simulink library "sensor_conversion_blocks"  (R2025b)
settings: Solver=VariableStepAuto  StartTime=0.0  StopTime=10.0  RelTol=1e-3
undefined symbols (not defined in the file): D
libraries: slrealtimeloglib x7, dspsigattribs x6, dspstat3 x5, dspfdesign x4, dspswit3 x2, eeGeneralControl x1
settings Model: Creator=cmmcguir  LastModifiedBy=cmmcguir

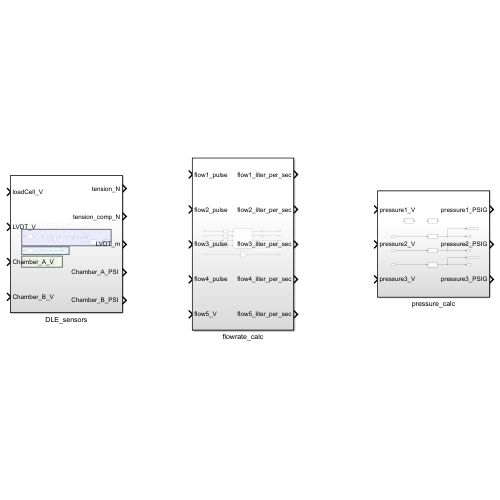
[thumbnail: Simulink's stored preview of the top-level diagram]
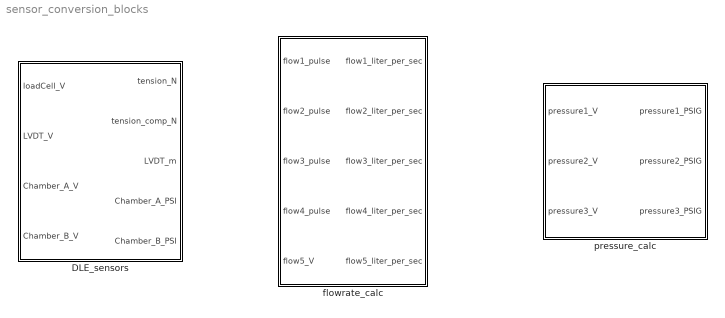
== system sensor_conversion_blocks ==
  DLE_sensors : Subsystem
  flowrate_calc : Subsystem
  pressure_calc : Subsystem

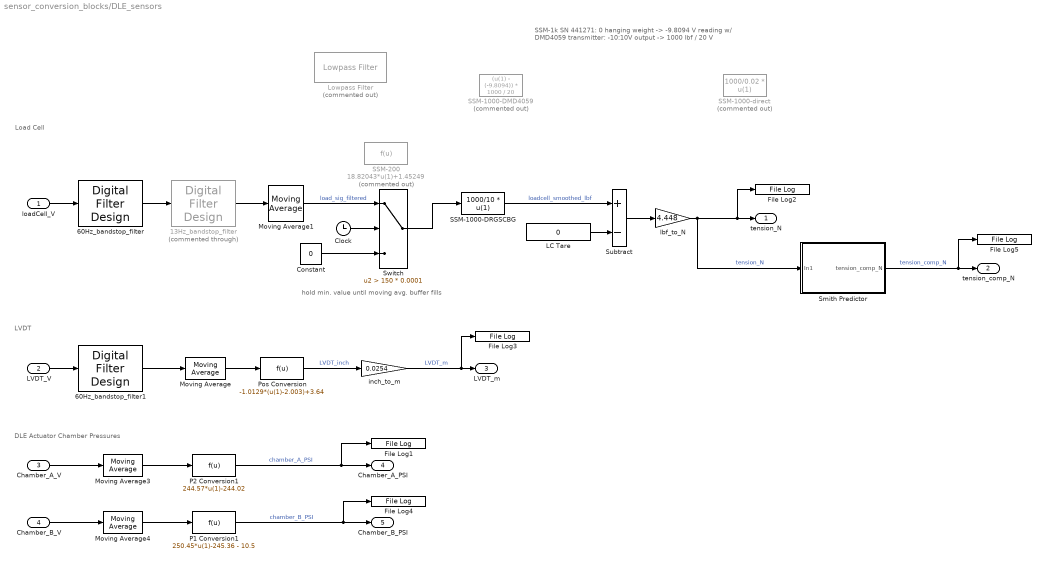
== system sensor_conversion_blocks/DLE_sensors ==
  note: hold min. value until moving avg. buffer fills
  note: SSM-1k SN 441271: 0 hanging weight -> -9.8094 V reading
      | w/ DMD4059 transmitter: -10:10V output -> 1000 lbf  / 20 V
  note: DLE Actuator Chamber Pressures
  note: LVDT
  note: Load Cell
  loadCell_V : Inport
  LVDT_V : Inport  Port=2
  Chamber_A_V : Inport  Port=3
  Chamber_B_V : Inport  Port=4
  13Hz_bandstop_filter : dspfdesign/Digital Filter Design  Commented=through  mwdsp_browser_bugfix_var=off
  60Hz_bandstop_filter : dspfdesign/Digital Filter Design  mwdsp_browser_bugfix_var=off
  60Hz_bandstop_filter1 : dspfdesign/Digital Filter Design  mwdsp_browser_bugfix_var=off
  Clock : Clock
  Constant : Constant  Value=0
  File Log{1..5} (5 alike) : slrealtimeloglib/File Log  decimation=1  inputProcessing=Elements as channels (sample based)
  LC Tare : Constant  Value=0
  Lowpass Filter : dspfdesign/Lowpass Filter  Commented=on  FilterType=FIR  DesignForMinimumOrder=on  FilterOrder=50  PassbandFrequency=10  StopbandFrequency=250  PassbandRipple=0.1  StopbandAttenuation=80  SampleRateMode=Specify on dialog  SampleRate=10000  SimulateUsing=Interpreted execution  roundingMode=Floor  coeffsDataTypeStr=fixdt(1,16)
  Moving Average : dspstat3/Moving Average  Method=Sliding window  ForgettingFactorPort=off  SpecifyWindowLength=on  WindowLength=150  OverlapLength=149  AllowArbitraryInputLength=off  ForgettingFactor=0.1  SimulateUsing=Code generation
  Moving Average1 : dspstat3/Moving Average  Method=Sliding window  ForgettingFactorPort=off  SpecifyWindowLength=on  WindowLength=150  OverlapLength=149  AllowArbitraryInputLength=off  ForgettingFactor=0.9  SimulateUsing=Interpreted execution
  Moving Average3 : dspstat3/Moving Average  Method=Sliding window  ForgettingFactorPort=off  SpecifyWindowLength=on  WindowLength=100  OverlapLength=99  AllowArbitraryInputLength=off  ForgettingFactor=0.1  SimulateUsing=Code generation
  Moving Average4 : dspstat3/Moving Average  Method=Sliding window  ForgettingFactorPort=off  SpecifyWindowLength=on  WindowLength=100  OverlapLength=99  AllowArbitraryInputLength=off  ForgettingFactor=0.1  SimulateUsing=Code generation
  P1 Conversion1 : Fcn  Expr=250.45*u(1)-245.36 - 10.5
  P2 Conversion1 : Fcn  Expr=244.57*u(1)-244.02
  Pos Conversion : Fcn  Expr=-1.0129*(u(1)-2.003)+3.64
  SSM-1000-DMD4059 : Fcn  Commented=on  Expr=(u(1) - (-9.8094)) * 1000 / 20
  SSM-1000-DRGSCBG : Fcn  Expr=1000/10 * u(1)
  SSM-1000-direct : Fcn  Commented=on  Expr=1000/0.02 * u(1)
  SSM-200 : Fcn  Commented=on  Expr=18.82043*u(1)+1.45249
  Smith Predictor : Subsystem
  Subtract : Sum  Inputs=+-
  Switch : Switch  Criteria=u2 > Threshold  Threshold=150 * 0.0001  SaturateOnIntegerOverflow=off  InputSameDT=off
  inch_to_m : Gain  Gain=0.0254
  lbf_to_N : Gain  Gain=4.448
  tension_N : Outport
  tension_comp_N : Outport  Port=2
  LVDT_m : Outport  Port=3
  "Chamber_A_PSI " : Outport  Port=4  VectorParamsAs1DForOutWhenUnconnected=off
  "Chamber_B_PSI " : Outport  Port=5  VectorParamsAs1DForOutWhenUnconnected=off
  wires:
  SSM-1000-DRGSCBG/1 -> Subtract/1  "loadcell_smoothed_lbf"
  LC Tare/1 -> Subtract/2
  Subtract/1 -> lbf_to_N/1
  lbf_to_N/1 -> Smith Predictor/1(In1), File Log2/1, tension_N/1  "tension_N"
  Pos Conversion/1 -> inch_to_m/1  "LVDT_inch"
  inch_to_m/1 -> File Log3/1, LVDT_m/1  "LVDT_m"
  60Hz_bandstop_filter/1 -> 13Hz_bandstop_filter/1
  13Hz_bandstop_filter/1 -> Moving Average1/1
  LVDT_V/1 -> 60Hz_bandstop_filter1/1
  60Hz_bandstop_filter1/1 -> Moving Average/1
  Moving Average/1 -> Pos Conversion/1
  P2 Conversion1/1 -> File Log1/1, "Chamber_A_PSI "/1  "chamber_A_PSI"
  P1 Conversion1/1 -> File Log4/1, "Chamber_B_PSI "/1  "chamber_B_PSI"
  Chamber_B_V/1 -> Moving Average4/1
  Chamber_A_V/1 -> Moving Average3/1
  Moving Average3/1 -> P2 Conversion1/1
  Moving Average4/1 -> P1 Conversion1/1
  Smith Predictor/1(tension_comp_N) -> File Log5/1, tension_comp_N/1  "tension_comp_N"
  Switch/1 -> SSM-1000-DRGSCBG/1
  Clock/1 -> Switch/2
  Constant/1 -> Switch/3
  loadCell_V/1 -> 60Hz_bandstop_filter/1
  Moving Average1/1 -> Switch/1  "load_sig_filtered"

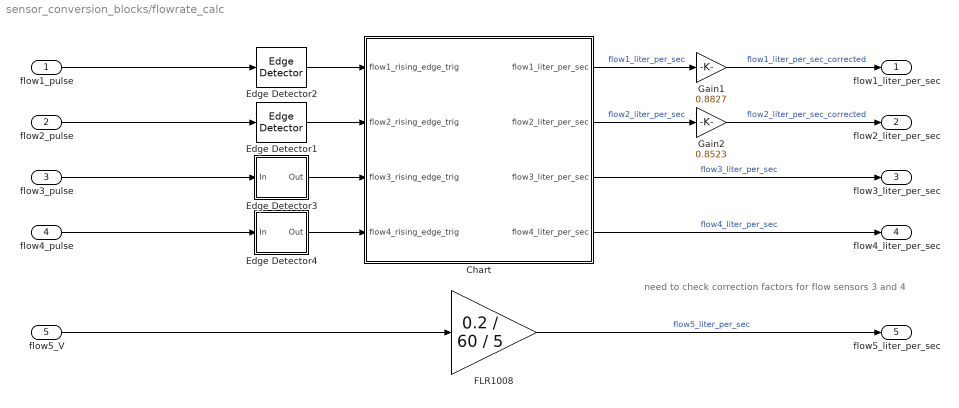
== system sensor_conversion_blocks/flowrate_calc ==
  note: need to check correction factors for flow sensors 3 and 4
  flow1_pulse : Inport
  flow2_pulse : Inport  Port=2
  flow3_pulse : Inport  Port=3
  flow4_pulse : Inport  Port=4
  flow5_V : Inport  Port=5
  Chart : Stateflow chart  TreatAsAtomicUnit=on
  Edge Detector1 : dspswit3/Edge Detector  InputProcessing=Columns as channels (frame based)
  Edge Detector2 : dspswit3/Edge Detector  InputProcessing=Columns as channels (frame based)
  Edge Detector3 : Subsystem  mask(Edge Detector){InputProcessing=Columns as channels (frame based)}
      mask prompts: InputProcessing "dsp:FIRMultirateBlockDialog:InputProc_MP"
      mask help: dsp:DSPSwitchesBlockDialog:EdgeDetector_MaskDesc
      mask init:
      | inputProc = get_param(gcbh, 'InputProcessing');
      | set_param([gcb '/Delay'], 'InputProcessing', inputProc);
      mask Help: eval('blocksethelp');
      mask TypeOptions InputProcessing: dsp:dialog:InProcessingFrameBased_CB | dsp:dialog:InProcessingSampleBased_CB
      mask DialogControl InputProcessing Prompt: Input processing:
      mask Display:
      | x = [.1 .2 .2 .5 .5 .7 .7 .8 .8 .9 NaN .1 .9 NaN .2 .2 NaN .7 .7];
      | y = [.6 .6 .9 .9 .6 .6 .9 .9 .6 .6 NaN .1 .1 NaN .1 .5 NaN .1 .5];
      | plot(x,y)
  Edge Detector4 : Subsystem  mask(Edge Detector){InputProcessing=Columns as channels (frame based)}
      mask prompts: InputProcessing "dsp:FIRMultirateBlockDialog:InputProc_MP"
      mask help: dsp:DSPSwitchesBlockDialog:EdgeDetector_MaskDesc
      mask init:
      | inputProc = get_param(gcbh, 'InputProcessing');
      | set_param([gcb '/Delay'], 'InputProcessing', inputProc);
      mask Help: eval('blocksethelp');
      mask TypeOptions InputProcessing: dsp:dialog:InProcessingFrameBased_CB | dsp:dialog:InProcessingSampleBased_CB
      mask DialogControl InputProcessing Prompt: Input processing:
      mask Display:
      | x = [.1 .2 .2 .5 .5 .7 .7 .8 .8 .9 NaN .1 .9 NaN .2 .2 NaN .7 .7];
      | y = [.6 .6 .9 .9 .6 .6 .9 .9 .6 .6 NaN .1 .1 NaN .1 .5 NaN .1 .5];
      | plot(x,y)
  FLR1008 : Gain  Gain=0.2 / 60 / 5
  Gain1 : Gain  Gain=0.8827
  Gain2 : Gain  Gain=0.8523
  flow1_liter_per_sec : Outport
  flow2_liter_per_sec : Outport  Port=2
  flow3_liter_per_sec : Outport  Port=3
  flow4_liter_per_sec : Outport  Port=4
  flow5_liter_per_sec : Outport  Port=5
  wires:
  flow2_pulse/1 -> Edge Detector1/1
  Edge Detector1/1 -> Chart/2(flow2_rising_edge_trig)
  Chart/1(flow1_liter_per_sec) -> Gain1/1  "flow1_liter_per_sec"
  Chart/2(flow2_liter_per_sec) -> Gain2/1  "flow2_liter_per_sec"
  flow1_pulse/1 -> Edge Detector2/1
  Edge Detector2/1 -> Chart/1(flow1_rising_edge_trig)
  Gain1/1 -> flow1_liter_per_sec/1  "flow1_liter_per_sec_corrected"
  Gain2/1 -> flow2_liter_per_sec/1  "flow2_liter_per_sec_corrected"
  flow3_pulse/1 -> Edge Detector3/1(In)
  flow4_pulse/1 -> Edge Detector4/1(In)
  Edge Detector3/1(Out) -> Chart/3(flow3_rising_edge_trig)
  Edge Detector4/1(Out) -> Chart/4(flow4_rising_edge_trig)
  Chart/3(flow3_liter_per_sec) -> flow3_liter_per_sec/1  "flow3_liter_per_sec"
  Chart/4(flow4_liter_per_sec) -> flow4_liter_per_sec/1  "flow4_liter_per_sec"
  flow5_V/1 -> FLR1008/1
  FLR1008/1 -> flow5_liter_per_sec/1  "flow5_liter_per_sec"

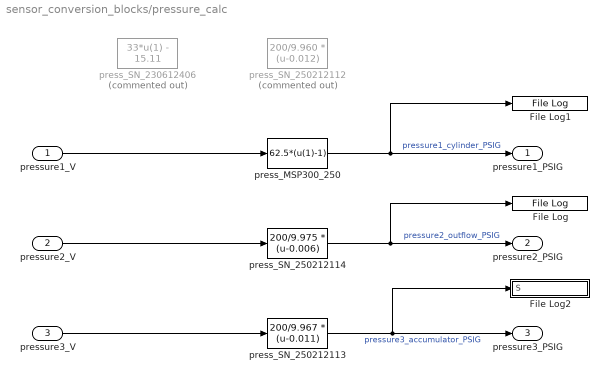
== system sensor_conversion_blocks/pressure_calc ==
  pressure1_V : Inport
  pressure2_V : Inport  Port=2
  pressure3_V : Inport  Port=3
  File Log : slrealtimeloglib/File Log  decimation=1  inputProcessing=Elements as channels (sample based)
  File Log1 : slrealtimeloglib/File Log  decimation=1  inputProcessing=Elements as channels (sample based)
  File Log2 : Subsystem  mask(slrealtimeloggingblock){decimation=1, inputProcessing=Elements as channels (sample based)}
      mask prompts: decimation "slrealtime:maskStrings:Decimation"; inputProcessing "slrealtime:maskStrings:InputProcessing"
      mask help: slrealtime:maskStrings:FileLogDesc
      mask init:
      | slrealtime.internal.logging.mloggingblock(gcb, decimation, inputProcessing);
      mask Help: eval('slrealtimedoc(''File_Log'')');
      mask TypeOptions inputProcessing: slrealtime:maskStrings:FrameBased | slrealtime:maskStrings:SampleBased
      mask DialogControl DescGroupVar Prompt: File Log
      mask DialogControl decimation Prompt: Decimation
      mask DialogControl inputProcessing Prompt: Input Processing
      mask Display: fprintf(message('slrealtime:maskStrings:FileLogDisp').getString);
  press_MSP300_250 : Fcn  Expr=62.5*(u(1)-1)
  press_SN_230612406 : Fcn  Commented=on  Expr=33*u(1) - 15.11
  press_SN_250212112 : Fcn  Commented=on  Expr=200/9.960 * (u-0.012)
  press_SN_250212113 : Fcn  Expr=200/9.967 * (u-0.011)
  press_SN_250212114 : Fcn  Expr=200/9.975 * (u-0.006)
  pressure1_PSIG : Outport
  pressure2_PSIG : Outport  Port=2
  pressure3_PSIG : Outport  Port=3
  wires:
  pressure1_V/1 -> press_MSP300_250/1
  press_MSP300_250/1 -> pressure1_PSIG/1, File Log1/1  "pressure1_cylinder_PSIG"
  press_SN_250212114/1 -> pressure2_PSIG/1, File Log/1  "pressure2_outflow_PSIG"
  pressure2_V/1 -> press_SN_250212114/1
  pressure3_V/1 -> press_SN_250212113/1
  press_SN_250212113/1 -> File Log2/1(S), pressure3_PSIG/1  "pressure3_accumulator_PSIG"

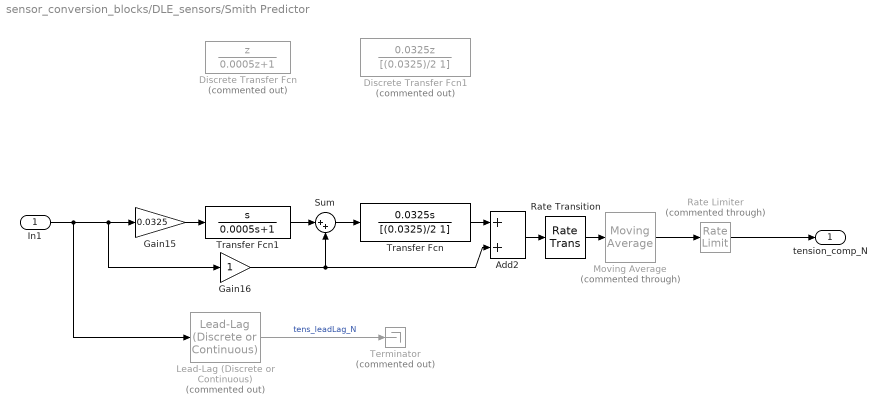
== system sensor_conversion_blocks/DLE_sensors/Smith Predictor ==
  In1 : Inport
  Add2 : Sum
  Discrete Transfer Fcn : DiscreteTransferFcn  Commented=on  Numerator=[1 0]  Denominator=[0.0005 1]
  Discrete Transfer Fcn1 : DiscreteTransferFcn  Commented=on  Numerator=[0.0325 0]  Denominator=[(0.0325)/2 1]
  Gain15 : Gain  Gain=0.0325
  Gain16 : Gain
  Lead-Lag (Discrete or Continuous) : eeGeneralControl/Lead-Lag (Discrete or Continuous)  Commented=on  T1=0.3  T2=0.1  B=inf  A=-inf  init_option=Inherited from block input  x0=0  Ts=-1
      settings: LibrarySourceBlock=|
      | ee_sl_lib/General Control/Lead-Lag
      | (Discrete or Continuous)
  Moving Average : dspstat3/Moving Average  Commented=through  Method=Sliding window  ForgettingFactorPort=off  SpecifyWindowLength=on  WindowLength=50  OverlapLength=49  AllowArbitraryInputLength=off  ForgettingFactor=0.9  SimulateUsing=Interpreted execution
  Rate Limiter : RateLimiter  Commented=through  RisingSlewLimit=4e3  FallingSlewLimit=-4e3  SampleTimeMode=inherited
  Rate Transition : RateTransition  OutPortSampleTime=0.0001
  Sum : Sum  Inputs=|++
  Terminator : Terminator  Commented=on
  Transfer Fcn : TransferFcn  Numerator=[0.0325 0]  Denominator=[(0.0325)/2 1]
  Transfer Fcn1 : TransferFcn  Numerator=[1 0]  Denominator=[0.0005 1]
  tension_comp_N : Outport
  wires:
  Gain16/1 -> Sum/2, Add2/2
  Transfer Fcn1/1 -> Sum/1
  In1/1 -> Lead-Lag (Discrete or Continuous)/1, Gain15/1, Gain16/1
  Gain15/1 -> Transfer Fcn1/1
  Add2/1 -> Rate Transition/1
  Sum/1 -> Transfer Fcn/1
  Transfer Fcn/1 -> Add2/1
  Moving Average/1 -> Rate Limiter/1
  Rate Transition/1 -> Moving Average/1
  Lead-Lag (Discrete or Continuous)/1 -> Terminator/1  "tens_leadLag_N"
  Rate Limiter/1 -> tension_comp_N/1

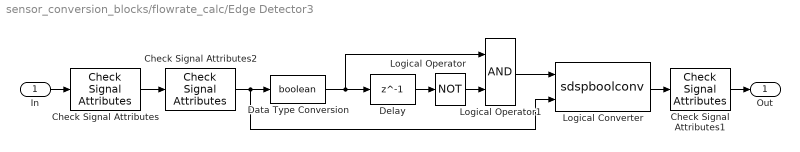
== system sensor_conversion_blocks/flowrate_calc/Edge Detector3 ==
  In : Inport
  Check Signal Attributes : dspsigattribs/Check Signal Attributes  SigAttribCheckMethod=Matches attributes exactly  Complexity=Ignore  Frame=Ignore  DimsCheckMethod=Ignore  Dimensions=1-D  DatatypeCheckMethod=Is...  DatatypeGeneral=Enumerated  DtypeFloatSpecific=Any floating-point  DtypeFixedSpecific=Any fixed-point  DtypeIntSpecific=Any integer  SampleMode=Ignore
  Check Signal Attributes1 : dspsigattribs/Check Signal Attributes  SigAttribCheckMethod=Matches attributes exactly  Complexity=Ignore  Frame=Ignore  DimsCheckMethod=Ignore  Dimensions=1-D  DatatypeCheckMethod=Is...  DatatypeGeneral=Enumerated  DtypeFloatSpecific=Any floating-point  DtypeFixedSpecific=Any fixed-point  DtypeIntSpecific=Any integer  SampleMode=Ignore
  Check Signal Attributes2 : dspsigattribs/Check Signal Attributes  SigAttribCheckMethod=Matches attributes exactly  Complexity=Ignore  Frame=Ignore  DimsCheckMethod=Ignore  Dimensions=1-D  DatatypeCheckMethod=Ignore  DatatypeGeneral=Enumerated  DtypeFloatSpecific=Any floating-point  DtypeFixedSpecific=Any fixed-point  DtypeIntSpecific=Any integer  SampleMode=Continuous
  Data Type Conversion : DataTypeConversion  OutDataTypeStr=boolean
  Delay : Delay  DelayLength=1  InitialCondition=1  InputProcessing=Columns as channels (frame based)
  Logical Operator : Logic  Operator=NOT  Inputs=1
  Logical Operator1 : Logic
  Logical Converter : S-Function  FunctionName=sdspboolconv  SFunctionDeploymentMode=off  EnableBusSupport=off
      mask Display:
      | disp('Logical\nConverter');
      | 
      | 
      | 
      | 
      | 
      | port_label('input',1, 'In');
      | 
      | 
      | 
      | 
      | 
      | port_label('input',2, 'Ref');
  Out : Outport  InitialOutput=0
  wires:
  Logical Operator1/1 -> Logical Converter/1
  Logical Operator/1 -> Logical Operator1/2
  Data Type Conversion/1 -> Logical Operator1/1, Delay/1
  Delay/1 -> Logical Operator/1
  In/1 -> Check Signal Attributes/1
  Logical Converter/1 -> Check Signal Attributes1/1
  Check Signal Attributes/1 -> Check Signal Attributes2/1
  Check Signal Attributes1/1 -> Out/1
  Check Signal Attributes2/1 -> Logical Converter/2, Data Type Conversion/1

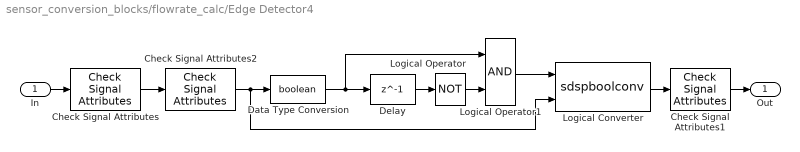
== system sensor_conversion_blocks/flowrate_calc/Edge Detector4 ==
  In : Inport
  Check Signal Attributes : dspsigattribs/Check Signal Attributes  SigAttribCheckMethod=Matches attributes exactly  Complexity=Ignore  Frame=Ignore  DimsCheckMethod=Ignore  Dimensions=1-D  DatatypeCheckMethod=Is...  DatatypeGeneral=Enumerated  DtypeFloatSpecific=Any floating-point  DtypeFixedSpecific=Any fixed-point  DtypeIntSpecific=Any integer  SampleMode=Ignore
  Check Signal Attributes1 : dspsigattribs/Check Signal Attributes  SigAttribCheckMethod=Matches attributes exactly  Complexity=Ignore  Frame=Ignore  DimsCheckMethod=Ignore  Dimensions=1-D  DatatypeCheckMethod=Is...  DatatypeGeneral=Enumerated  DtypeFloatSpecific=Any floating-point  DtypeFixedSpecific=Any fixed-point  DtypeIntSpecific=Any integer  SampleMode=Ignore
  Check Signal Attributes2 : dspsigattribs/Check Signal Attributes  SigAttribCheckMethod=Matches attributes exactly  Complexity=Ignore  Frame=Ignore  DimsCheckMethod=Ignore  Dimensions=1-D  DatatypeCheckMethod=Ignore  DatatypeGeneral=Enumerated  DtypeFloatSpecific=Any floating-point  DtypeFixedSpecific=Any fixed-point  DtypeIntSpecific=Any integer  SampleMode=Continuous
  Data Type Conversion : DataTypeConversion  OutDataTypeStr=boolean
  Delay : Delay  DelayLength=1  InitialCondition=1  InputProcessing=Columns as channels (frame based)
  Logical Operator : Logic  Operator=NOT  Inputs=1
  Logical Operator1 : Logic
  Logical Converter : S-Function  FunctionName=sdspboolconv  SFunctionDeploymentMode=off  EnableBusSupport=off
      mask Display:
      | disp('Logical\nConverter');
      | 
      | 
      | 
      | 
      | 
      | port_label('input',1, 'In');
      | 
      | 
      | 
      | 
      | 
      | port_label('input',2, 'Ref');
  Out : Outport  InitialOutput=0
  wires:
  Check Signal Attributes2/1 -> Data Type Conversion/1, Logical Converter/2
  Check Signal Attributes1/1 -> Out/1
  Check Signal Attributes/1 -> Check Signal Attributes2/1
  Logical Converter/1 -> Check Signal Attributes1/1
  In/1 -> Check Signal Attributes/1
  Delay/1 -> Logical Operator/1
  Data Type Conversion/1 -> Delay/1, Logical Operator1/1
  Logical Operator/1 -> Logical Operator1/2
  Logical Operator1/1 -> Logical Converter/1

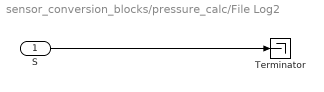
== system sensor_conversion_blocks/pressure_calc/File Log2 ==
  S : Inport
  Terminator : Terminator
  wires:
  S/1 -> Terminator/1

== stateflow chart sensor_conversion_blocks/flowrate_calc/Chart ==
  state flow1 [parallel]
    settings: executionOrder=1
    state wait1
      en:
      flow1_period = t - flow1_timestamp;
      flow1_liter_per_sec = 1 / (flow1_period * ft110_pulse_per_liter);
      flow1_timestamp = t;
    state sensor1_idle
      en:
      flow1_liter_per_sec = 0;
    (junction 24) -> wait1
    (junction 23) -> (junction 24)
    wait1 -> sensor1_idle [order 2] : [after(1.2*flow1_period, sec)]
    wait1 -> (junction 22) [order 1] : [flow1_rising_edge_trig]
    (junction 22) -> (junction 23)
    (default) -> sensor1_idle
    (junction 42) -> (junction 23)
    sensor1_idle -> (junction 42) : [flow1_rising_edge_trig]
  state flow2 [parallel]
    settings: executionOrder=2
    state wait2
      en:
      flow2_period = t - flow2_timestamp;
      flow2_liter_per_sec = 1 / (flow2_period * ft110_pulse_per_liter);
      flow2_timestamp = t;
    state sensor2_idle
      en:
      flow2_liter_per_sec = 0;
    (junction 54) -> wait2
    (junction 50) -> (junction 54)
    wait2 -> sensor2_idle [order 2] : [after(1.2*flow2_period, sec)]
    wait2 -> (junction 46) [order 1] : [flow2_rising_edge_trig]
    (junction 46) -> (junction 50)
    (default) -> sensor2_idle
    (junction 57) -> (junction 50)
    sensor2_idle -> (junction 57) : [flow2_rising_edge_trig]
  state flow3 [parallel]
    settings: executionOrder=3
    state wait3
      en:
      flow3_period = t - flow3_timestamp;
      flow3_liter_per_sec = 1 / (flow3_period * ft110_pulse_per_liter);
      flow3_timestamp = t;
    state sensor3_idle
      en:
      flow3_liter_per_sec = 0;
    (junction 73) -> wait3
    (junction 69) -> (junction 73)
    wait3 -> sensor3_idle [order 2] : [after(1.2*flow3_period, sec)]
    wait3 -> (junction 68) [order 1] : [flow3_rising_edge_trig]
    (junction 68) -> (junction 69)
    (default) -> sensor3_idle
    (junction 79) -> (junction 69)
    sensor3_idle -> (junction 79) : [flow3_rising_edge_trig]
  state flow4 [parallel]
    settings: executionOrder=4
    state wait4
      en:
      flow4_period = t - flow4_timestamp;
      flow4_liter_per_sec = 1 / (flow4_period * ft210_pulse_per_liter);
      flow4_timestamp = t;
    state sensor4_idle
      en:
      flow4_liter_per_sec = 0;
    (junction 94) -> wait4
    (junction 87) -> (junction 94)
    wait4 -> sensor4_idle [order 2] : [after(1.2*flow4_period, sec)]
    wait4 -> (junction 92) [order 1] : [flow4_rising_edge_trig]
    (junction 92) -> (junction 87)
    (default) -> sensor4_idle
    (junction 96) -> (junction 87)
    sensor4_idle -> (junction 96) : [flow4_rising_edge_trig]
  data: flow1_rising_edge_trig input; flow2_rising_edge_trig input; ft110_pulse_per_liter local =4700; flow1_liter_per_sec output =0; flow2_liter_per_sec output =0; flow1_timestamp local =0; flow2_timestamp local =0; flow1_period local =0; flow2_period local =0; flow3_rising_edge_trig input; flow3_liter_per_sec output =0; flow3_timestamp local =0; flow3_period local =0; flow4_rising_edge_trig input; flow4_liter_per_sec output =0; flow4_timestamp local =0; flow4_period local =0; ft210_pulse_per_liter local =83200/3.785
